simulink model "gofa"  (R2024b)
settings: Solver=FixedStepAuto  StartTime=0.0  StopTime=38.48  FixedStep=0.001  RelTol=1e-3
undefined symbols (not defined in the file or in its folder): X, Y, Z
libraries: sm_lib x69, nesl_utility x7
(part 2 of 2)

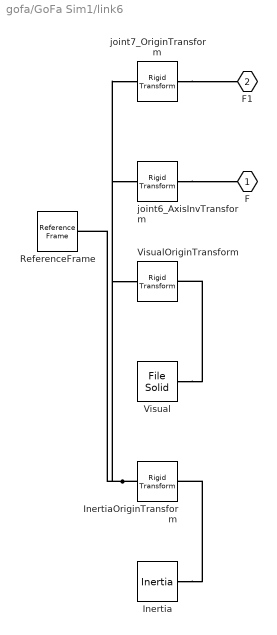
== system gofa/GoFa Sim1/link6 ==
  Inertia : sm_lib/Body Elements/Inertia  InertiaType=Custom  Mass=2  MassUnits=kg  CenterOfMass=[0, 0, 0]  CenterOfMassUnits=m  MomentsOfInertia=[10, 10, 10]  MomentsOfInertiaUnits=kg*m^2  ProductsOfInertia=[0, 0, 0]  ProductsOfInertiaUnits=kg*m^2  GraphicType=None  MarkerShape=Inertia  MarkerSize=20  GraphicVisPropType=SimpleVisualProperties  GraphicDiffuseColor=[0.5 0.5 0.5]  GraphicOpacity=1  GraphicSpecularColor=[0.5 0.5 0.5 1.0]  GraphicAmbientColor=[0.15 0.15 0.15 1.0]  GraphicEmissiveColor=[0.0 0.0 0.0 1.0]  GraphicShininess=75
  InertiaOriginTransform : sm_lib/Frames and Transforms/Rigid Transform  RotationMethod=RotationSequence  FollAlignAxisA=+X  BaseAlignAxisA=+Y  FollAlignAxisB=+Y  BaseAlignAxisB=+Z  RotationStandardAxis=+Z  RotationAngle=0  RotationAngleUnits=deg  RotationArbitraryAxis=[0 0 1]  RotationSequenceAxes=BaseAxes  RotationSequence=XYZ  RotationSequenceAngles=[0, 0, 0]  RotationSequenceAnglesUnits=rad  RotationMatrix=[1 0 0;0 1 0;0 0 1]  Quaternion=[1 0 0 0]  TranslationMethod=Cartesian  TranslationCartesianOffset=[0, 0, 0]  TranslationCartesianOffsetUnits=m  TranslationStandardAxis=+Z  TranslationStandardOffset=0  TranslationStandardOffsetUnits=m  TranslationROffset=0  TranslationROffsetUnits=m  TranslationThetaOffset=0  TranslationThetaOffsetUnits=deg  TranslationZOffset=0  TranslationZOffsetUnits=m
  ReferenceFrame : sm_lib/Frames and Transforms/Reference Frame
  Visual : sm_lib/Body Elements/File Solid  ExtGeomFileName=link6.STL  UnitType=Custom  ExtGeomFileUnits=m  StepReaderType=HEX  ExportConvexHullGeometry=off  InertiaType=Custom  BasedOnType=DensityFromFile  Density=1000  DensityUnits=kg/m^3  Mass=0  MassUnits=kg  CenterOfMass=[0, 0, 0]  CenterOfMassUnits=m  MomentsOfInertia=[0, 0, 0]  MomentsOfInertiaUnits=kg*m^2  ProductsOfInertia=[0, 0, 0]  ProductsOfInertiaUnits=kg*m^2  GraphicType=FromGeometry  MarkerShape=Sphere  MarkerSize=10  GraphicVisPropType=SimpleVisualProperties  GraphicDiffuseColor=[0.83, 0.83, 0.83]  GraphicOpacity=1  GraphicSpecularColor=[0.5 0.5 0.5 1.0]  GraphicAmbientColor=[0.15 0.15 0.15 1.0]  GraphicEmissiveColor=[0.0 0.0 0.0 1.0]  GraphicShininess=75  DoExposeReferenceFrame=on  SerializedFrames=<Frames/>
  VisualOriginTransform : sm_lib/Frames and Transforms/Rigid Transform  RotationMethod=RotationSequence  FollAlignAxisA=+X  BaseAlignAxisA=+Y  FollAlignAxisB=+Y  BaseAlignAxisB=+Z  RotationStandardAxis=+Z  RotationAngle=0  RotationAngleUnits=deg  RotationArbitraryAxis=[0 0 1]  RotationSequenceAxes=BaseAxes  RotationSequence=XYZ  RotationSequenceAngles=[0, 0, 0]  RotationSequenceAnglesUnits=rad  RotationMatrix=[1 0 0;0 1 0;0 0 1]  Quaternion=[1 0 0 0]  TranslationMethod=Cartesian  TranslationCartesianOffset=[0, 0, 0]  TranslationCartesianOffsetUnits=m  TranslationStandardAxis=+Z  TranslationStandardOffset=0  TranslationStandardOffsetUnits=m  TranslationROffset=0  TranslationROffsetUnits=m  TranslationThetaOffset=0  TranslationThetaOffsetUnits=deg  TranslationZOffset=0  TranslationZOffsetUnits=m
  joint6_AxisInvTransform : sm_lib/Frames and Transforms/Rigid Transform  RotationMethod=ArbitraryAxis  FollAlignAxisA=+X  BaseAlignAxisA=+Y  FollAlignAxisB=+Y  BaseAlignAxisB=+Z  RotationStandardAxis=+Z  RotationAngle=0  RotationAngleUnits=rad  RotationArbitraryAxis=[1, 0, 0]  RotationSequenceAxes=FollowerAxes  RotationSequence=XYX  RotationSequenceAngles=[0 0 0]  RotationSequenceAnglesUnits=deg  RotationMatrix=[1 0 0;0 1 0;0 0 1]  Quaternion=[1 0 0 0]  TranslationMethod=Cartesian  TranslationCartesianOffset=[0, 0, 0]  TranslationCartesianOffsetUnits=m  TranslationStandardAxis=+Z  TranslationStandardOffset=0  TranslationStandardOffsetUnits=m  TranslationROffset=0  TranslationROffsetUnits=m  TranslationThetaOffset=0  TranslationThetaOffsetUnits=deg  TranslationZOffset=0  TranslationZOffsetUnits=m
  joint7_OriginTransform : sm_lib/Frames and Transforms/Rigid Transform  RotationMethod=RotationSequence  FollAlignAxisA=+X  BaseAlignAxisA=+Y  FollAlignAxisB=+Y  BaseAlignAxisB=+Z  RotationStandardAxis=+Z  RotationAngle=0  RotationAngleUnits=deg  RotationArbitraryAxis=[0 0 1]  RotationSequenceAxes=BaseAxes  RotationSequence=XYZ  RotationSequenceAngles=[1.5708, -1.5708, 0]  RotationSequenceAnglesUnits=rad  RotationMatrix=[1 0 0;0 1 0;0 0 1]  Quaternion=[1 0 0 0]  TranslationMethod=Cartesian  TranslationCartesianOffset=[0, -0.1527, 0.1261]  TranslationCartesianOffsetUnits=m  TranslationStandardAxis=+Z  TranslationStandardOffset=0  TranslationStandardOffsetUnits=m  TranslationROffset=0  TranslationROffsetUnits=m  TranslationThetaOffset=0  TranslationThetaOffsetUnits=deg  TranslationZOffset=0  TranslationZOffsetUnits=m
  F : PMIOPort  Side=Left
  F1 : PMIOPort  Port=2  Side=Right
  connections:
  Inertia/RConn1 -- InertiaOriginTransform/RConn1
  ReferenceFrame/RConn1 -- InertiaOriginTransform/LConn1 -- VisualOriginTransform/LConn1 -- joint6_AxisInvTransform/LConn1 -- joint7_OriginTransform/LConn1
  Visual/RConn1 -- VisualOriginTransform/RConn1
  joint6_AxisInvTransform/RConn1 -- F/RConn1
  joint7_OriginTransform/RConn1 -- F1/RConn1

== matlab function gofa/GoFa kinematic ==
  data: x output; t1 input; y output; t2 input; t3 input; t4 input; t5 input; t6 input; z output; R output
function [x,y,z,R] = fcn(t1,t2,t3,t4,t5,t6)

% Constant params
% d3= 0.15;
% a2 = 0.4318;
% a3 = 0.0203;
% d4 = 0.4318;
% d5 = 0.1;

% end effector position
x = (444*cos(t1)*cos(t2) + (3997*cos(t5)*(sin(t1)*sin(t4) - cos(t4)*(cos(t1)*sin(t2)*sin(t3) - cos(t1)*cos(t2)*cos(t3))))/50 - (3818*cos(t6)*(cos(t4)*sin(t1) + sin(t4)*(cos(t1)*sin(t2)*sin(t3) - cos(t1)*cos(t2)*cos(t3))))/25 + (389*sin(t5)*(sin(t1)*sin(t4) - cos(t4)*(cos(t1)*sin(t2)*sin(t3) - cos(t1)*cos(t2)*cos(t3))))/2 + (3818*sin(t6)*(cos(t5)*(sin(t1)*sin(t4) - cos(t4)*(cos(t1)*sin(t2)*sin(t3) - cos(t1)*cos(t2)*cos(t3))) - sin(t5)*(cos(t1)*cos(t2)*sin(t3) + cos(t1)*cos(t3)*sin(t2))))/25 + (389*cos(t5)*(cos(t1)*cos(t2)*sin(t3) + cos(t1)*cos(t3)*sin(t2)))/2 - (3997*sin(t5)*(cos(t1)*cos(t2)*sin(t3) + cos(t1)*cos(t3)*sin(t2)))/50 - 110*cos(t1)*sin(t2)*sin(t3) + 110*cos(t1)*cos(t2)*cos(t3) + 470*cos(t1)*cos(t2)*sin(t3) + 470*cos(t1)*cos(t3)*sin(t2))/1000;

y = (444*cos(t2)*sin(t1) - (3997*cos(t5)*(cos(t1)*sin(t4) + cos(t4)*(sin(t1)*sin(t2)*sin(t3) - cos(t2)*cos(t3)*sin(t1))))/50 + (3818*cos(t6)*(cos(t1)*cos(t4) - sin(t4)*(sin(t1)*sin(t2)*sin(t3) - cos(t2)*cos(t3)*sin(t1))))/25 - (389*sin(t5)*(cos(t1)*sin(t4) + cos(t4)*(sin(t1)*sin(t2)*sin(t3) - cos(t2)*cos(t3)*sin(t1))))/2 + (389*cos(t5)*(cos(t2)*sin(t1)*sin(t3) + cos(t3)*sin(t1)*sin(t2)))/2 - (3818*sin(t6)*(cos(t5)*(cos(t1)*sin(t4) + cos(t4)*(sin(t1)*sin(t2)*sin(t3) - cos(t2)*cos(t3)*sin(t1))) + sin(t5)*(cos(t2)*sin(t1)*sin(t3) + cos(t3)*sin(t1)*sin(t2))))/25 - (3997*sin(t5)*(cos(t2)*sin(t1)*sin(t3) + cos(t3)*sin(t1)*sin(t2)))/50 + 470*cos(t2)*sin(t1)*sin(t3) + 470*cos(t3)*sin(t1)*sin(t2) - 110*sin(t1)*sin(t2)*sin(t3) + 110*cos(t2)*cos(t3)*sin(t1))/1000;

z = (444*sin(t2) - 470*cos(t2)*cos(t3) + 110*cos(t2)*sin(t3) + 110*cos(t3)*sin(t2) + 470*sin(t2)*sin(t3) + (3818*sin(t6)*(sin(t5)*(cos(t2)*cos(t3) - sin(t2)*sin(t3)) + cos(t4)*cos(t5)*(cos(t2)*sin(t3) + cos(t3)*sin(t2))))/25 - (389*cos(t5)*(cos(t2)*cos(t3) - sin(t2)*sin(t3)))/2 + (3997*sin(t5)*(cos(t2)*cos(t3) - sin(t2)*sin(t3)))/50 + (3997*cos(t4)*cos(t5)*(cos(t2)*sin(t3) + cos(t3)*sin(t2)))/50 + (389*cos(t4)*sin(t5)*(cos(t2)*sin(t3) + cos(t3)*sin(t2)))/2 + (3818*cos(t6)*sin(t4)*(cos(t2)*sin(t3) + cos(t3)*sin(t2)))/25 + 263)/1000;

r_matrix = zeros(3,3);

r_matrix(1,1) = sin(t5)*(sin(t1)*sin(t4) - cos(t4)*(cos(t1)*sin(t2)*sin(t3) - cos(t1)*cos(t2)*cos(t3))) + cos(t5)*(cos(t1)*cos(t2)*sin(t3) + cos(t1)*cos(t3)*sin(t2));

r_matrix(1,2) = -sin(t6)*(cos(t4)*sin(t1) + sin(t4)*(cos(t1)*sin(t2)*sin(t3) - cos(t1)*cos(t2)*cos(t3))) - cos(t6)*(cos(t5)*(sin(t1)*sin(t4) - cos(t4)*(cos(t1)*sin(t2)*sin(t3) - cos(t1)*cos(t2)*cos(t3))) - sin(t5)*(cos(t1)*cos(t2)*sin(t3) + cos(t1)*cos(t3)*sin(t2)));

r_matrix(1,3) = sin(t6)*(cos(t5)*(sin(t1)*sin(t4) - cos(t4)*(cos(t1)*sin(t2)*sin(t3) - cos(t1)*cos(t2)*cos(t3))) - sin(t5)*(cos(t1)*cos(t2)*sin(t3) + cos(t1)*cos(t3)*sin(t2))) - cos(t6)*(cos(t4)*sin(t1) + sin(t4)*(cos(t1)*sin(t2)*sin(t3) - cos(t1)*cos(t2)*cos(t3)));

r_matrix(2,1) =  cos(t5)*(cos(t2)*sin(t1)*sin(t3) + cos(t3)*sin(t1)*sin(t2)) - sin(t5)*(cos(t1)*sin(t4) + cos(t4)*(sin(t1)*sin(t2)*sin(t3) - cos(t2)*cos(t3)*sin(t1)));

r_matrix(2,2) = sin(t6)*(cos(t1)*cos(t4) - sin(t4)*(sin(t1)*sin(t2)*sin(t3) - cos(t2)*cos(t3)*sin(t1))) + cos(t6)*(cos(t5)*(cos(t1)*sin(t4) + cos(t4)*(sin(t1)*sin(t2)*sin(t3) - cos(t2)*cos(t3)*sin(t1))) + sin(t5)*(cos(t2)*sin(t1)*sin(t3) + cos(t3)*sin(t1)*sin(t2)));

r_matrix(2,3) = cos(t6)*(cos(t1)*cos(t4) - sin(t4)*(sin(t1)*sin(t2)*sin(t3) - cos(t2)*cos(t3)*sin(t1))) - sin(t6)*(cos(t5)*(cos(t1)*sin(t4) + cos(t4)*(sin(t1)*sin(t2)*sin(t3) - cos(t2)*cos(t3)*sin(t1))) + sin(t5)*(cos(t2)*sin(t1)*sin(t3) + cos(t3)*sin(t1)*sin(t2)));

r_matrix(3,1) =cos(t4)*sin(t5)*(cos(t2)*sin(t3) + cos(t3)*sin(t2)) - cos(t5)*(cos(t2)*cos(t3) - sin(t2)*sin(t3));

r_matrix(3,2) = sin(t4)*sin(t6)*(cos(t2)*sin(t3) + cos(t3)*sin(t2)) - cos(t6)*(sin(t5)*(cos(t2)*cos(t3) - sin(t2)*sin(t3)) + cos(t4)*cos(t5)*(cos(t2)*sin(t3) + cos(t3)*sin(t2)));

r_matrix(3,3) = sin(t6)*(sin(t5)*(cos(t2)*cos(t3) - sin(t2)*sin(t3)) + cos(t4)*cos(t5)*(cos(t2)*sin(t3) + cos(t3)*sin(t2))) + cos(t6)*sin(t4)*(cos(t2)*sin(t3) + cos(t3)*sin(t2));

R = r_matrix;

== matlab function gofa/Inverse Jacobian ==
  settings: updateMethod=DISCRETE
  data: dx input; output_joint_value output; dy input; dz input; d_alpha input; d_beta input; d_gamma input; joint_value input; output_djoint_value output; det_J output
% function [dt1,dt2,dt3,dt4,dt5,dt6] = fcn(dx,dy,dz,d_alpha,d_beta,d_gamma, joint_value)
function [output_joint_value,output_djoint_value,det_J]  = fcn(dx,dy,dz,d_alpha,d_beta,d_gamma, joint_value)
% persistent theta1 theta2 theta3 theta4 theta5 theta6
% if isempty(theta1)
%     theta1 =  1e-5;
%     theta2 =  1e-5;
%     theta3 =  1e-5;
%     theta4 =  1e-5;
%     theta5 =  1e-5;
%     theta6 =  1e-5;    
% end

% constant parameters
d3= 0.15;
a2 = 0.4318;
a3 = 0.0203;
d4 = 0.4318;
d5 = 0.1;
dt =0.01;

if (length(joint_value)>1)
    t1 = joint_value(1);
    t2 = joint_value(2);
    t3 = joint_value(3);
    t4 = joint_value(4);
    t5 = joint_value(5);
    t6 = joint_value(6);
else
    t1 =  1e-5;
    t2 =  1e-5;
    t3 =  1e-5;
    t4 =  1e-5;
    t5 =  1e-5;
    t6 =  1e-5;
end

j_matrix = zeros(6,6);

j_matrix(1,1) = ((3997*cos(t5)*(cos(t1)*sin(t4) + cos(t4)*(sin(t1)*sin(t2)*sin(t3) - cos(t2)*cos(t3)*sin(t1))))/50 - 444*cos(t2)*sin(t1) - (3818*cos(t6)*(cos(t1)*cos(t4) - sin(t4)*(sin(t1)*sin(t2)*sin(t3) - cos(t2)*cos(t3)*sin(t1))))/25 + (389*sin(t5)*(cos(t1)*sin(t4) + cos(t4)*(sin(t1)*sin(t2)*sin(t3) - cos(t2)*cos(t3)*sin(t1))))/2 - (389*cos(t5)*(cos(t2)*sin(t1)*sin(t3) + cos(t3)*sin(t1)*sin(t2)))/2 + (3818*sin(t6)*(cos(t5)*(cos(t1)*sin(t4) + cos(t4)*(sin(t1)*sin(t2)*sin(t3) - cos(t2)*cos(t3)*sin(t1))) + sin(t5)*(cos(t2)*sin(t1)*sin(t3) + cos(t3)*sin(t1)*sin(t2))))/25 + (3997*sin(t5)*(cos(t2)*sin(t1)*sin(t3) + cos(t3)*sin(t1)*sin(t2)))/50 - 470*cos(t2)*sin(t1)*sin(t3) - 470*cos(t3)*sin(t1)*sin(t2) + 110*sin(t1)*sin(t2)*sin(t3) - 110*cos(t2)*cos(t3)*sin(t1))/1000;

j_matrix(1,2) = (-(cos(t1)*(22200*sin(t2) - 23500*cos(t2)*cos(t3) + 5500*cos(t2)*sin(t3) + 5500*cos(t3)*sin(t2) + 23500*sin(t2)*sin(t3) - 9725*cos(t2 + t3)*cos(t5) + 3997*cos(t2 + t3)*sin(t5) + 3997*sin(t2 + t3)*cos(t4)*cos(t5) + 9725*sin(t2 + t3)*cos(t4)*sin(t5) + 7636*sin(t2 + t3)*cos(t6)*sin(t4) + 7636*cos(t2 + t3)*sin(t5)*sin(t6) + 7636*sin(t2 + t3)*cos(t4)*cos(t5)*sin(t6)))/50)/1000;

j_matrix(1,3) = (-(cos(t1)*(5500*cos(t2)*sin(t3) - 23500*cos(t2)*cos(t3) + 5500*cos(t3)*sin(t2) + 23500*sin(t2)*sin(t3) - 9725*cos(t2 + t3)*cos(t5) + 3997*cos(t2 + t3)*sin(t5) + 3997*sin(t2 + t3)*cos(t4)*cos(t5) + 9725*sin(t2 + t3)*cos(t4)*sin(t5) + 7636*sin(t2 + t3)*cos(t6)*sin(t4) + 7636*cos(t2 + t3)*sin(t5)*sin(t6) + 7636*sin(t2 + t3)*cos(t4)*cos(t5)*sin(t6)))/50)/1000;

j_matrix(1,4) = ((3997*cos(t5)*(cos(t4)*sin(t1) + sin(t4)*(cos(t1)*sin(t2)*sin(t3) - cos(t1)*cos(t2)*cos(t3))))/50 + (3818*cos(t6)*(sin(t1)*sin(t4) - cos(t4)*(cos(t1)*sin(t2)*sin(t3) - cos(t1)*cos(t2)*cos(t3))))/25 + (389*sin(t5)*(cos(t4)*sin(t1) + sin(t4)*(cos(t1)*sin(t2)*sin(t3) - cos(t1)*cos(t2)*cos(t3))))/2 + (3818*cos(t5)*sin(t6)*(cos(t4)*sin(t1) + sin(t4)*(cos(t1)*sin(t2)*sin(t3) - cos(t1)*cos(t2)*cos(t3))))/25)/1000;

j_matrix(1,5) = ((389*cos(t5)*(sin(t1)*sin(t4) - cos(t4)*(cos(t1)*sin(t2)*sin(t3) - cos(t1)*cos(t2)*cos(t3))))/2 - (3997*sin(t5)*(sin(t1)*sin(t4) - cos(t4)*(cos(t1)*sin(t2)*sin(t3) - cos(t1)*cos(t2)*cos(t3))))/50 - (3818*sin(t6)*(sin(t5)*(sin(t1)*sin(t4) - cos(t4)*(cos(t1)*sin(t2)*sin(t3) - cos(t1)*cos(t2)*cos(t3))) + cos(t5)*(cos(t1)*cos(t2)*sin(t3) + cos(t1)*cos(t3)*sin(t2))))/25 - (3997*cos(t5)*(cos(t1)*cos(t2)*sin(t3) + cos(t1)*cos(t3)*sin(t2)))/50 - (389*sin(t5)*(cos(t1)*cos(t2)*sin(t3) + cos(t1)*cos(t3)*sin(t2)))/2)/1000;

j_matrix(1,6) = ((3818*sin(t6)*(cos(t4)*sin(t1) + sin(t4)*(cos(t1)*sin(t2)*sin(t3) - cos(t1)*cos(t2)*cos(t3))))/25 + (3818*cos(t6)*(cos(t5)*(sin(t1)*sin(t4) - cos(t4)*(cos(t1)*sin(t2)*sin(t3) - cos(t1)*cos(t2)*cos(t3))) - sin(t5)*(cos(t1)*cos(t2)*sin(t3) + cos(t1)*cos(t3)*sin(t2))))/25)/1000;

j_matrix(2,1) = (444*cos(t1)*cos(t2) + (3997*cos(t5)*(sin(t1)*sin(t4) - cos(t4)*(cos(t1)*sin(t2)*sin(t3) - cos(t1)*cos(t2)*cos(t3))))/50 - (3818*cos(t6)*(cos(t4)*sin(t1) + sin(t4)*(cos(t1)*sin(t2)*sin(t3) - cos(t1)*cos(t2)*cos(t3))))/25 + (389*sin(t5)*(sin(t1)*sin(t4) - cos(t4)*(cos(t1)*sin(t2)*sin(t3) - cos(t1)*cos(t2)*cos(t3))))/2 + (3818*sin(t6)*(cos(t5)*(sin(t1)*sin(t4) - cos(t4)*(cos(t1)*sin(t2)*sin(t3) - cos(t1)*cos(t2)*cos(t3))) - sin(t5)*(cos(t1)*cos(t2)*sin(t3) + cos(t1)*cos(t3)*sin(t2))))/25 + (389*cos(t5)*(cos(t1)*cos(t2)*sin(t3) + cos(t1)*cos(t3)*sin(t2)))/2 - (3997*sin(t5)*(cos(t1)*cos(t2)*sin(t3) + cos(t1)*cos(t3)*sin(t2)))/50 - 110*cos(t1)*sin(t2)*sin(t3) + 110*cos(t1)*cos(t2)*cos(t3) + 470*cos(t1)*cos(t2)*sin(t3) + 470*cos(t1)*cos(t3)*sin(t2))/1000;

j_matrix(2,2) = (-(sin(t1)*(22200*sin(t2) - 23500*cos(t2)*cos(t3) + 5500*cos(t2)*sin(t3) + 5500*cos(t3)*sin(t2) + 23500*sin(t2)*sin(t3) - 9725*cos(t2 + t3)*cos(t5) + 3997*cos(t2 + t3)*sin(t5) + 3997*sin(t2 + t3)*cos(t4)*cos(t5) + 9725*sin(t2 + t3)*cos(t4)*sin(t5) + 7636*sin(t2 + t3)*cos(t6)*sin(t4) + 7636*cos(t2 + t3)*sin(t5)*sin(t6) + 7636*sin(t2 + t3)*cos(t4)*cos(t5)*sin(t6)))/50)/1000;

j_matrix(2,3) = (-(sin(t1)*(5500*cos(t2)*sin(t3) - 23500*cos(t2)*cos(t3) + 5500*cos(t3)*sin(t2) + 23500*sin(t2)*sin(t3) - 9725*cos(t2 + t3)*cos(t5) + 3997*cos(t2 + t3)*sin(t5) + 3997*sin(t2 + t3)*cos(t4)*cos(t5) + 9725*sin(t2 + t3)*cos(t4)*sin(t5) + 7636*sin(t2 + t3)*cos(t6)*sin(t4) + 7636*cos(t2 + t3)*sin(t5)*sin(t6) + 7636*sin(t2 + t3)*cos(t4)*cos(t5)*sin(t6)))/50)/1000;

j_matrix(2,4) = (- (3997*cos(t5)*(cos(t1)*cos(t4) - sin(t4)*(sin(t1)*sin(t2)*sin(t3) - cos(t2)*cos(t3)*sin(t1))))/50 - (3818*cos(t6)*(cos(t1)*sin(t4) + cos(t4)*(sin(t1)*sin(t2)*sin(t3) - cos(t2)*cos(t3)*sin(t1))))/25 - (389*sin(t5)*(cos(t1)*cos(t4) - sin(t4)*(sin(t1)*sin(t2)*sin(t3) - cos(t2)*cos(t3)*sin(t1))))/2 - (3818*cos(t5)*sin(t6)*(cos(t1)*cos(t4) - sin(t4)*(sin(t1)*sin(t2)*sin(t3) - cos(t2)*cos(t3)*sin(t1))))/25)/1000;

j_matrix(2,5) = ((3997*sin(t5)*(cos(t1)*sin(t4) + cos(t4)*(sin(t1)*sin(t2)*sin(t3) - cos(t2)*cos(t3)*sin(t1))))/50 - (389*cos(t5)*(cos(t1)*sin(t4) + cos(t4)*(sin(t1)*sin(t2)*sin(t3) - cos(t2)*cos(t3)*sin(t1))))/2 - (3997*cos(t5)*(cos(t2)*sin(t1)*sin(t3) + cos(t3)*sin(t1)*sin(t2)))/50 + (3818*sin(t6)*(sin(t5)*(cos(t1)*sin(t4) + cos(t4)*(sin(t1)*sin(t2)*sin(t3) - cos(t2)*cos(t3)*sin(t1))) - cos(t5)*(cos(t2)*sin(t1)*sin(t3) + cos(t3)*sin(t1)*sin(t2))))/25 - (389*sin(t5)*(cos(t2)*sin(t1)*sin(t3) + cos(t3)*sin(t1)*sin(t2)))/2)/1000;

j_matrix(2,6) = (- (3818*sin(t6)*(cos(t1)*cos(t4) - sin(t4)*(sin(t1)*sin(t2)*sin(t3) - cos(t2)*cos(t3)*sin(t1))))/25 - (3818*cos(t6)*(cos(t5)*(cos(t1)*sin(t4) + cos(t4)*(sin(t1)*sin(t2)*sin(t3) - cos(t2)*cos(t3)*sin(t1))) + sin(t5)*(cos(t2)*sin(t1)*sin(t3) + cos(t3)*sin(t1)*sin(t2))))/25)/1000;

j_matrix(3,1) = 0;

j_matrix(3,2) = (110*cos(t2 + t3) + 470*sin(t2 + t3) + 444*cos(t2) - (3997*sin(t2 + t3)*sin(t5))/50 + (3997*cos(t4 - t5)*cos(t2 + t3))/100 - (389*sin(t4 - t5)*cos(t2 + t3))/4 + (1909*sin(t4 - t6)*cos(t2 + t3))/25 + (3997*cos(t2 + t3)*cos(t4 + t5))/100 + (389*cos(t2 + t3)*sin(t4 + t5))/4 + (1909*cos(t2 + t3)*sin(t4 + t6))/25 + (389*sin(t2 + t3)*cos(t5))/2 + (1909*cos(t2 + t3)*cos(t4 + t5)*sin(t6))/25 - (3818*sin(t2 + t3)*sin(t5)*sin(t6))/25 + (1909*cos(t4 - t5)*cos(t2 + t3)*sin(t6))/25)/1000;

j_matrix(3,3) = (110*cos(t2 + t3) + 470*sin(t2 + t3) - (3997*sin(t2 + t3)*sin(t5))/50 + (389*sin(t2 + t3)*cos(t5))/2 + (3997*cos(t2 + t3)*cos(t4)*cos(t5))/50 + (389*cos(t2 + t3)*cos(t4)*sin(t5))/2 + (3818*cos(t2 + t3)*cos(t6)*sin(t4))/25 - (3818*sin(t2 + t3)*sin(t5)*sin(t6))/25 + (3818*cos(t2 + t3)*cos(t4)*cos(t5)*sin(t6))/25)/1000;
j_matrix(3,4) = (-(sin(t2 + t3)*(3997*cos(t5)*sin(t4) - 7636*cos(t4)*cos(t6) + 9725*sin(t4)*sin(t5) + 7636*cos(t5)*sin(t4)*sin(t6)))/50)/1000;
j_matrix(3,5) = ((3818*sin(t6)*(cos(t2 + t3)*cos(t5) - sin(t2 + t3)*cos(t4)*sin(t5)))/25 + (3997*cos(t2 + t3)*cos(t5))/50 + (389*cos(t2 + t3)*sin(t5))/2 + (389*sin(t2 + t3)*cos(t4)*cos(t5))/2 - (3997*sin(t2 + t3)*cos(t4)*sin(t5))/50)/1000;
j_matrix(3,6) = ((3818*cos(t6)*(cos(t2 + t3)*sin(t5) + sin(t2 + t3)*cos(t4)*cos(t5)))/25 - (3818*sin(t2 + t3)*sin(t4)*sin(t6))/25)/1000;


j_matrix(4,1) = 0;
j_matrix(4,2) = sin(t1);
j_matrix(4,3) = sin(t1);
j_matrix(4,4) =  sin(t2 + t3)*cos(t1);
j_matrix(4,5) = cos(t4)*sin(t1) + sin(t4)*(cos(t1)*sin(t2)*sin(t3) - cos(t1)*cos(t2)*cos(t3));
j_matrix(4,6) = sin(t5)*(sin(t1)*sin(t4) - cos(t4)*(cos(t1)*sin(t2)*sin(t3) - cos(t1)*cos(t2)*cos(t3))) + cos(t5)*(cos(t1)*cos(t2)*sin(t3) + cos(t1)*cos(t3)*sin(t2));

j_matrix(5,1) = 0;
j_matrix(5,2) = -cos(t1);
j_matrix(5,3) = -cos(t1);
j_matrix(5,4) =  sin(t2 + t3)*sin(t1);
j_matrix(5,5) = sin(t4)*(sin(t1)*sin(t2)*sin(t3) - cos(t2)*cos(t3)*sin(t1)) - cos(t1)*cos(t4);
j_matrix(5,6) = cos(t5)*(cos(t2)*sin(t1)*sin(t3) + cos(t3)*sin(t1)*sin(t2)) - sin(t5)*(cos(t1)*sin(t4) + cos(t4)*(sin(t1)*sin(t2)*sin(t3) - cos(t2)*cos(t3)*sin(t1)));

j_matrix(6,1) = 1;
j_matrix(6,2) = 0;
j_matrix(6,3) = 0;
j_matrix(6,4) =  - cos(t2 + t3);
j_matrix(6,5) = -sin(t2 + t3)*sin(t4);
j_matrix(6,6) = sin(t2 + t3)*cos(t4)*sin(t5) - cos(t2 + t3)*cos(t5);

d_ef = [dx dy dz d_alpha d_beta d_gamma]';

% d_joint = inv(j_matrix)*d_ef;
d_joint = j_matrix\d_ef;


dt1 = d_joint(1);
dt2 = d_joint(2);
dt3 = d_joint(3);
dt4 = d_joint(4);
dt5 = d_joint(5);
dt6 = d_joint(6);


output_joint_value =zeros(6,1);

output_joint_value(1) = dt1 + t1;
output_joint_value(2) = dt2 + t2;
output_joint_value(3) = dt3 + t3;
output_joint_value(4) = dt4 + t4;
output_joint_value(5) = dt5 + t5;
output_joint_value(6) = dt6 + t6;

output_djoint_value =zeros(6,1);

output_djoint_value(1) = dt1;
output_djoint_value(2) = dt2;
output_djoint_value(3) = dt3;
output_djoint_value(4) = dt4;
output_djoint_value(5) = dt5;
output_djoint_value(6) = dt6;

% J = j_matrix;
det_J = det(j_matrix);
